simulink model "test_thrust"  (Simulink 7.7)
settings: Solver=ode45  StartTime=0.0  StopTime=10  RelTol=1e-3
settings Model: Creator=Administrator  LastModifiedBy=Administrator

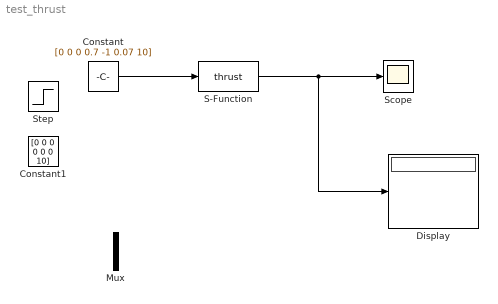
== system test_thrust ==
  Constant : Constant  Value=[0 0 0 0.7 -1 0.07 10]
  Constant1 : Constant  Value=[0 0 0 0 0 0 10]
  Display : Display
  Mux : Mux  Inputs=2
  S-Function : S-Function  FunctionName=thrust  EnableBusSupport=off
  Scope : Scope
  Step : Step  SampleTime=0
  wires:
  S-Function/1 -> Scope/1, Display/1
  Constant/1 -> S-Function/1
